simulink model "sampleModel37"  (R2021b)
settings: Solver=VariableStepAuto  StartTime=0.0  StopTime=10.0  RelTol=1e-3
libraries: simulink x4, slpidlib x1
settings Model: Creator=user  LastModifiedBy=user

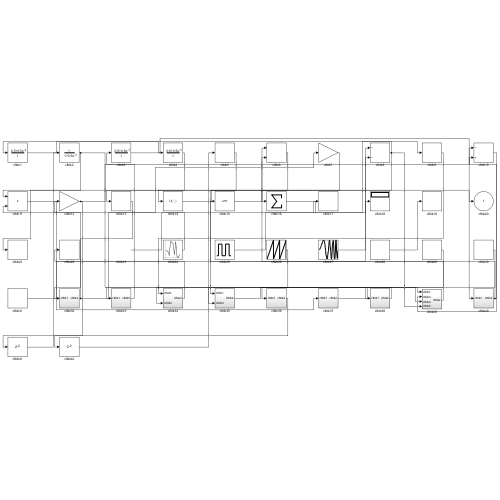
[thumbnail: Simulink's stored preview of the top-level diagram]
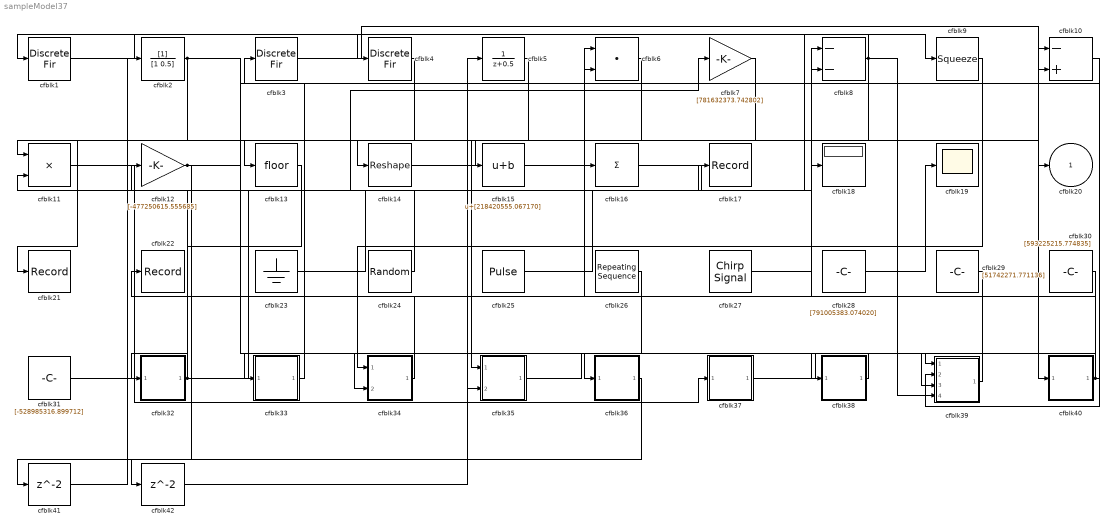
== system sampleModel37 ==
  cfblk1 : DiscreteFir  SampleTime=1
  cfblk10 : Sum  Inputs=-+
  cfblk11 : Product
  cfblk12 : Gain  Gain=[-477250615.555685]
  cfblk13 : Rounding
  cfblk14 : Reshape
  cfblk15 : Bias  Bias=[218420555.067170]
  cfblk16 : Sum  Inputs=+
  cfblk17 : Record  FileSettingsInternal="{\"entries\":[{\"content\":{\"excelSettings\":{\"content\":{},\"type\":\"Streamout.ExcelSettings\"}},\"type\":\"Streamout.FileSettingStorage\",\"uuid\":\"7168dcdb-680c-4d2a-a763-12b65a08ef9c\"}],\"packageUris\":[\"http://schema.mathworks.com/mf0/streamout_blocks/R2020a\"],\"version\":\"1.0\"}"  SignalsInternal="{\"entries\":[{\"content\":{\"signals\":[{\"content\":{\"blockPath\":[\"sampleModel37/cfblk17\"],\"channel\":[],\"dimensions\":[1],\"domain\":\"sampleModel37/cfblk17\",\"lineColor\":\"#ff6929\",\"plots\":[1],\"port\":1,\"sid\":[\"\"],\"signalID\":1459,\"signalName\":\"cfblk25\"},\"type\":\"RecordBlkView.Signal\",\"uuid\":\"e61bde02-3dd6-4be1-9ad0-feaebe9eeaeb\"}]},\"type\":\"RecordBlkView.InputSignals\",\"uuid\":\"cdbd18a7-85fd-4cfd-94b4-7f03027b774d\"}],\"packageUris\":[\"http://schema.mathworks.com/mf0/streamout_blocks/R2020a\"],\"version\":\"1.0\"}"  VisualizationBindings="{\"sparklinesplugin\":{\"info\":[{\"bindingParametersList\":[],\"subplotID\":1}]}}"
  cfblk18 : Display
  cfblk19 : Scope
  cfblk2 : DiscreteFilter  SampleTime=1
  cfblk21 : Record  FileSettingsInternal="{\"entries\":[{\"content\":{\"excelSettings\":{\"content\":{},\"type\":\"Streamout.ExcelSettings\"}},\"type\":\"Streamout.FileSettingStorage\",\"uuid\":\"b01cac01-9860-4d12-b080-a0c4ad3a2659\"}],\"packageUris\":[\"http://schema.mathworks.com/mf0/streamout_blocks/R2020a\"],\"version\":\"1.0\"}"  SignalsInternal="{\"entries\":[{\"content\":{\"signals\":[{\"content\":{\"blockPath\":[\"sampleModel37/cfblk21\"],\"channel\":[],\"dimensions\":[1],\"domain\":\"sampleModel37/cfblk21\",\"lineColor\":\"#139fff\",\"plots\":[1],\"port\":1,\"sid\":[\"\"],\"signalID\":1455,\"signalName\":\"cfblk4\"},\"type\":\"RecordBlkView.Signal\",\"uuid\":\"60c84040-f79e-415d-ad23-74debbbbaca6\"}]},\"type\":\"RecordBlkView.InputSignals\",\"uuid\":\"611b3d33-6149-406e-92cb-eac5bc08a6d0\"}],\"packageUris\":[\"http://schema.mathworks.com/mf0/streamout_blocks/R2020a\"],\"version\":\"1.0\"}"  VisualizationBindings="{\"sparklinesplugin\":{\"info\":[{\"bindingParametersList\":[],\"subplotID\":1}]}}"
  cfblk22 : Record  FileSettingsInternal="{\"entries\":[{\"content\":{\"excelSettings\":{\"content\":{},\"type\":\"Streamout.ExcelSettings\"}},\"type\":\"Streamout.FileSettingStorage\",\"uuid\":\"1630d272-9723-4f5e-9eaa-70344c1eee65\"}],\"packageUris\":[\"http://schema.mathworks.com/mf0/streamout_blocks/R2020a\"],\"version\":\"1.0\"}"  SignalsInternal="{\"entries\":[{\"content\":{\"signals\":[{\"content\":{\"blockPath\":[\"sampleModel37/cfblk22\"],\"channel\":[],\"dimensions\":[1],\"domain\":\"sampleModel37/cfblk22\",\"lineColor\":\"#b746ff\",\"plots\":[1],\"port\":1,\"sid\":[\"\"],\"signalID\":1463,\"signalName\":\"cfblk34\"},\"type\":\"RecordBlkView.Signal\",\"uuid\":\"da135b4a-7bbb-43f2-b09b-5a9c54f0beec\"}]},\"type\":\"RecordBlkView.InputSignals\",\"uuid\":\"8143830e-b97f-435e-a893-b43e763bd10a\"}],\"packageUris\":[\"http://schema.mathworks.com/mf0/streamout_blocks/R2020a\"],\"version\":\"1.0\"}"  VisualizationBindings="{\"sparklinesplugin\":{\"info\":[{\"bindingParametersList\":[],\"subplotID\":1}]}}"
  cfblk23 : Ground
  cfblk24 : RandomNumber  Mean=[26557.260662]  Variance=[75927.264061]  Seed=[233894079.000000]  SampleTime=0.1
  cfblk25 : DiscretePulseGenerator  PulseType=Time based  Amplitude=[-422549321.593864]  Period=[2269784.388946]  PulseWidth=5  PhaseDelay=[3.000000]
  cfblk26 : simulink/Sources/Repeating Sequence  rep_seq_t=[0 2]  rep_seq_y=[-291834772.823931, 299260622.817075]
  cfblk27 : simulink/Sources/Chirp Signal  f1=[215203401.127644]  T=[512335847.192583]  f2=[768727103.022336]
  cfblk28 : Constant  Value=[791005383.074020]  SampleTime=1
  cfblk29 : Constant  Value=[51742271.771136]  SampleTime=1
  cfblk3 : DiscreteFir  SampleTime=1
  cfblk30 : Constant  Value=[593225215.774835]  SampleTime=1
  cfblk31 : Constant  Value=[-528985316.899712]  SampleTime=1
  cfblk32 : Subsystem
  cfblk33 : Subsystem
  cfblk34 : Subsystem
  cfblk35 : Subsystem
  cfblk36 : Subsystem
  cfblk37 : Subsystem
  cfblk38 : Subsystem
  cfblk39 : Subsystem
  cfblk4 : DiscreteFir  SampleTime=1
  cfblk40 : Subsystem
  cfblk41 : Delay  SampleTime=1
  cfblk42 : Delay  SampleTime=1
  cfblk5 : DiscreteTransferFcn  SampleTime=1
  cfblk6 : DotProduct  InputSameDT=on  OutDataTypeStr=Inherit: Inherit via internal rule
  cfblk7 : Gain  Gain=[781632373.742802]
  cfblk8 : Sum  Inputs=--
  cfblk9 : Squeeze
  cfblk20 : Outport
  wires:
  cfblk12/1 -> cfblk10/2, cfblk42/1
  cfblk7/1 -> cfblk14/1
  cfblk9/1 -> cfblk34/1(cfblk1)
  cfblk11/1 -> cfblk37/1(cfblk1)
  cfblk32/1(cfblk2) -> cfblk7/1, cfblk12/1
  cfblk37/1(cfblk2) -> cfblk39/1(cfblk1)
  cfblk34/1(cfblk2) -> cfblk22/1
  cfblk38/1(cfblk2) -> cfblk36/1(cfblk1)
  cfblk27/1 -> cfblk8/1
  cfblk16/1 -> cfblk9/1
  cfblk29/1 -> cfblk33/1(cfblk1)
  cfblk31/1 -> cfblk8/2
  cfblk35/1(cfblk2) -> cfblk38/1(cfblk1)
  cfblk3/1 -> cfblk40/1(cfblk1)
  cfblk30/1 -> cfblk34/2(cfblk3)
  cfblk14/1 -> cfblk20/1
  cfblk2/1 -> cfblk11/1, cfblk39/3(cfblk4)
  cfblk5/1 -> cfblk13/1
  cfblk15/1 -> cfblk6/1
  cfblk6/1 -> cfblk35/1(cfblk1)
  cfblk23/1 -> cfblk18/1
  cfblk1/1 -> cfblk4/1
  cfblk13/1 -> cfblk32/1(cfblk1)
  cfblk28/1 -> cfblk19/1
  cfblk39/1(cfblk2) -> cfblk6/2
  cfblk26/1 -> cfblk35/2(cfblk4)
  cfblk25/1 -> cfblk17/1
  cfblk4/1 -> cfblk21/1
  cfblk8/1 -> cfblk16/1, cfblk1/1, cfblk39/4(cfblk5)
  cfblk33/1(cfblk2) -> cfblk3/1
  cfblk10/1 -> cfblk39/2(cfblk3)
  cfblk40/1(cfblk2) -> cfblk15/1, cfblk10/1
  cfblk24/1 -> cfblk11/2
  cfblk36/1(cfblk2) -> cfblk41/1
  cfblk41/1 -> cfblk2/1
  cfblk42/1 -> cfblk5/1

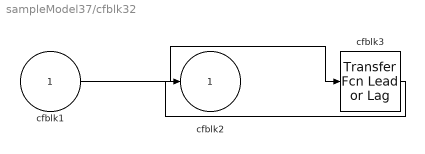
== system sampleModel37/cfblk32 ==
  cfblk1 : Inport
  cfblk3 : simulink/Discrete/Transfer Fcn Lead or Lag  PoleZ=0.95  ZeroZ=0.75  ICPrevOutput=0.0  ICPrevInput=0.0  DoSatur=off
      settings: SourceProductBaseCode=SL
  cfblk2 : Outport
  wires:
  cfblk1/1 -> cfblk3/1
  cfblk3/1 -> cfblk2/1

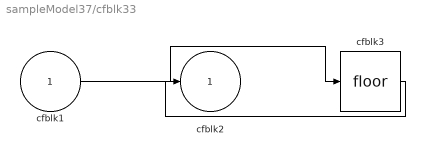
== system sampleModel37/cfblk33 ==
  cfblk1 : Inport
  cfblk3 : Rounding
  cfblk2 : Outport
  wires:
  cfblk1/1 -> cfblk3/1
  cfblk3/1 -> cfblk2/1

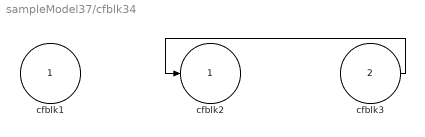
== system sampleModel37/cfblk34 ==
  cfblk1 : Inport
  cfblk3 : Inport  Port=2
  cfblk2 : Outport
  wires:
  cfblk3/1 -> cfblk2/1

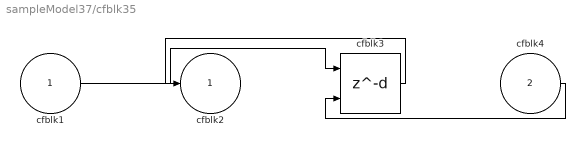
== system sampleModel37/cfblk35 ==
  cfblk1 : Inport
  cfblk4 : Inport  Port=2
  cfblk3 : Delay  DelayLengthSource=Input port  SampleTime=1
      settings: InputPortMap=u0,p1
  cfblk2 : Outport
  wires:
  cfblk1/1 -> cfblk3/1
  cfblk4/1 -> cfblk3/2
  cfblk3/1 -> cfblk2/1

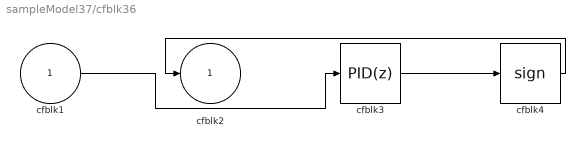
== system sampleModel37/cfblk36 ==
  cfblk1 : Inport
  cfblk3 : slpidlib/PID Controller  Controller=PID  Form=Parallel  TimeDomain=Discrete-time  UseExternalTs=off  SampleTime=1  IntegratorMethod=Forward Euler  FilterMethod=Forward Euler  ControllerParametersSource=internal  P=1  I=1  D=0  UseFilter=on  N=100  TunerSelectOption=Transfer Function Based (PID Tuner App)  InitialConditionSource=internal  InitialConditionForIntegrator=0  InitialConditionForFilter=0  DifferentiatorICPrevScaledInput=0  ExternalReset=none  TrackingMode=off  Kt=1  LimitOutput=off  SatLimitsSource=internal  UpperSaturationLimit=inf  LowerSaturationLimit=-inf  LinearizeAsGain=off  AntiWindupMode=none  Kb=1  POutMin=[]  POutMax=[]  IOutMin=[]  IOutMax=[]  DOutMin=[]  DOutMax=[]  NOutMin=[]  NOutMax=[]  SumOutMin=[]  SumOutMax=[]  SaturationOutMin=[]  SaturationOutMax=[]  PParamMin=[]  PParamMax=[]  IParamMin=[]  IParamMax=[]  DParamMin=[]  DParamMax=[]  NParamMin=[]  NParamMax=[]  KbParamMin=[]  KbParamMax=[]  KtParamMin=[]  KtParamMax=[]  KbOutMin=[]  KbOutMax=[]  KtOutMin=[]  KtOutMax=[]  IntegratorOutMin=[]  IntegratorOutMax=[]  FilterOutMin=[]  FilterOutMax=[]  SumI1OutMin=[]  SumI1OutMax=[]  SumI2OutMin=[]  SumI2OutMax=[]  SumI3OutMin=[]  SumI3OutMax=[]  SumI4OutMin=[]  SumI4OutMax=[]  SumDOutMin=[]  SumDOutMax=[]  DifferentiatorOutMin=[]  DifferentiatorOutMax=[]  FilterDiffOutCoefMin=[]  FilterDiffOutCoefMax=[]  ReciprocalOutMin=[]  ReciprocalOutMax=[]  SumDenOutMin=[]  SumDenOutMax=[]  SumNumOutMin=[]  SumNumOutMax=[]  DivideOutMin=[]  DivideOutMax=[]  UdiffTsProdOutMin=[]  UdiffTsProdOutMax=[]  NTsProdOutMin=[]  NTsProdOutMax=[]  UintegralTsProdOutMin=[]  UintegralTsProdOutMax=[]  UngainTsProdOutMin=[]  UngainTsProdOutMax=[]  IntegratorContinuousStateAttributes=''  IntegratorStateMustResolveToSignalObject=off  IntegratorRTWStateStorageClass=Auto  FilterContinuousStateAttributes=''  FilterStateMustResolveToSignalObject=off  FilterRTWStateStorageClass=Auto  ParallelPVariant=InternalParameters  IdealPVariant=Disabled  IVariant=InternalParameters  DVariant=InternalParameters  IntegratorVariant=Discrete  SatVariant=Disabled  AWVariant=Passthrough  PCopyVariant=Disabled  TRVariant=Disabled  FdbkBlocksVariant=Forward  IdealPFdbkVariant=Disabled  SatFdbkVariant=Disabled  DerivativeFilterVariant=ForwardEulerFilter  NVariant=InternalParameters  NCopyVariant=Disabled  FilterICVariant=InternalICsFilter  IntegratorICVariant=InternalICs  ExternalResetVariant=Disabled  TRSumVariant=Passthrough  SumFdbkVariant=Disabled  SumVariant=Sum_PID  TsampFilterVariant=InternalTs  TsampNgainVariant=Passthrough  TsampIntegralVariant=Passthrough  ExternalSaturationOutDataTypeStr=Inherit: Same as second input
  cfblk4 : Signum
  cfblk2 : Outport
  wires:
  cfblk4/1 -> cfblk2/1
  cfblk1/1 -> cfblk3/1
  cfblk3/1 -> cfblk4/1

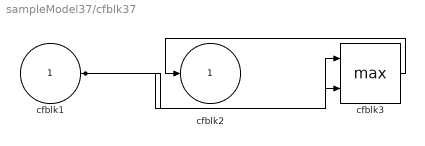
== system sampleModel37/cfblk37 ==
  cfblk1 : Inport
  cfblk3 : MinMax  Function=max  Inputs=2
  cfblk2 : Outport
  wires:
  cfblk3/1 -> cfblk2/1
  cfblk1/1 -> cfblk3/1, cfblk3/2

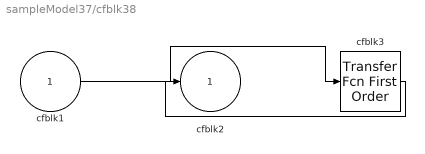
== system sampleModel37/cfblk38 ==
  cfblk1 : Inport
  cfblk3 : simulink/Discrete/Transfer Fcn First Order  PoleZ=0.95  ICPrevOutput=0.0  DoSatur=off
  cfblk2 : Outport
  wires:
  cfblk1/1 -> cfblk3/1
  cfblk3/1 -> cfblk2/1

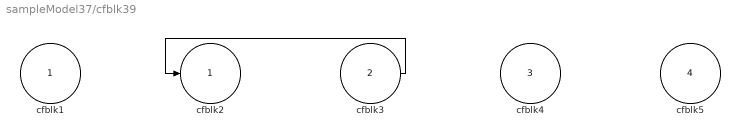
== system sampleModel37/cfblk39 ==
  cfblk1 : Inport
  cfblk3 : Inport  Port=2
  cfblk4 : Inport  Port=3
  cfblk5 : Inport  Port=4
  cfblk2 : Outport
  wires:
  cfblk3/1 -> cfblk2/1

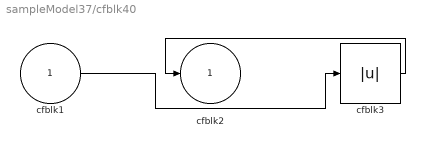
== system sampleModel37/cfblk40 ==
  cfblk1 : Inport
  cfblk3 : Abs
  cfblk2 : Outport
  wires:
  cfblk3/1 -> cfblk2/1
  cfblk1/1 -> cfblk3/1
